simulink model "Sim8s"  (R2014a)
settings: Solver=ode45  StartTime=0.0  StopTime=10.0  RelTol=1e-3
InitFcn:
  | V=1;
  | J=0.01;
  | b=0.1;
  | Ke=0.01;
  | Kt=0.07;
  | R=1;
  | L=0.5;
settings Model: Creator=OCAC  LastModifiedBy=OCAC

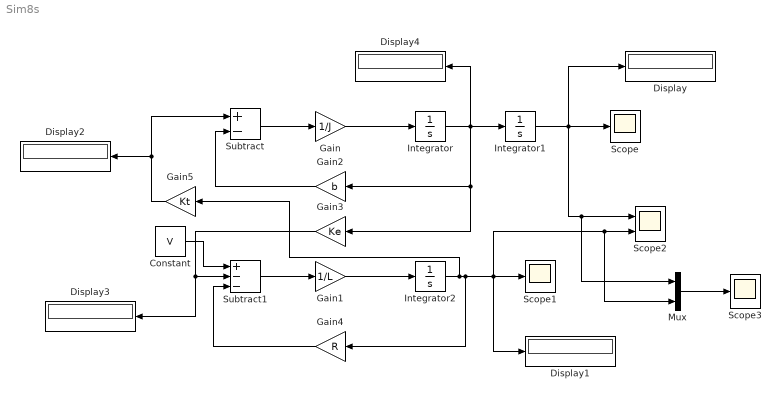
== system Sim8s ==
  Constant : Constant  Value=V
  Display{,1..4} (5 alike) : Display
  Gain : Gain  Gain=1/J
  Gain1 : Gain  Gain=1/L
  Gain2 : Gain  Gain=b
  Gain3 : Gain  Gain=Ke
  Gain4 : Gain  Gain=R
  Gain5 : Gain  Gain=Kt
  Integrator : Integrator
  Integrator1 : Integrator
  Integrator2 : Integrator
  Mux : Mux  Inputs=2
  Scope : Scope
  Scope1 : Scope
  Scope2 : Scope  NumInputPorts=2
      settings: YMin=-5~-5  YMax=5~5  SaveName=ScopeData2
  Scope3 : Scope
      settings: SaveName=ScopeData3
  Subtract : Sum  Inputs=+-
  Subtract1 : Sum  Inputs=+--
  wires:
  Subtract/1 -> Gain/1
  Gain/1 -> Integrator/1
  Integrator/1 -> Display4/1, Gain3/1, Gain2/1, Integrator1/1
  Constant/1 -> Subtract1/1
  Subtract1/1 -> Gain1/1
  Gain1/1 -> Integrator2/1
  Gain2/1 -> Subtract/2
  Gain3/1 -> Display3/1, Subtract1/2
  Gain4/1 -> Subtract1/3
  Integrator2/1 -> Display1/1, Mux/2, Scope2/2, Scope1/1, Gain4/1, Gain5/1
  Gain5/1 -> Display2/1, Subtract/1
  Integrator1/1 -> Display/1, Mux/1, Scope2/1, Scope/1
  Mux/1 -> Scope3/1
